simulink model "SensoresTEST"  (R2023b)
settings: Solver=VariableStepAuto  StartTime=0.0  StopTime=10.0  RelTol=1e-3
libraries: arduinolib x2
settings Model: Creator=Roberto  LastModifiedBy=Roberto

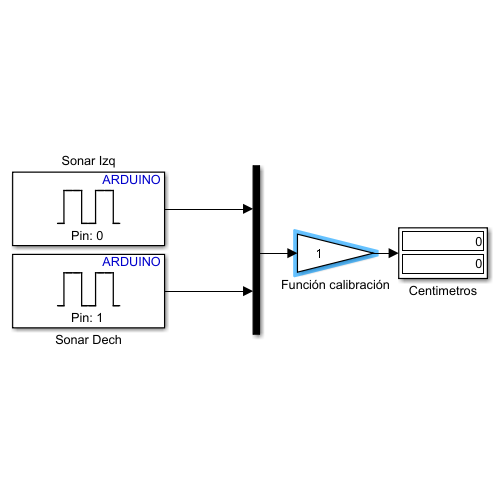
[thumbnail: Simulink's stored preview of the top-level diagram]
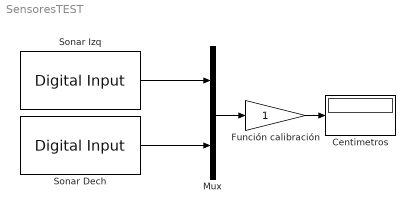
== system SensoresTEST ==
  Centimetros : Display
  Función calibración : Gain
  Mux : Mux  Inputs=2
  Sonar Dech : arduinolib/Digital Input  pinNumber=1  mode=Default  Direction=input  SampleTime=0.1  blockPlatform=arduino
  Sonar Izq : arduinolib/Digital Input  pinNumber=0  mode=Default  Direction=input  SampleTime=0.1  blockPlatform=arduino
  wires:
  Sonar Izq/1 -> Mux/1
  Sonar Dech/1 -> Mux/2
  Mux/1 -> Función calibración/1
  Función calibración/1 -> Centimetros/1
